simulink library "uavsimBlockset_Cularis_withUAV3D"  (Simulink 8.6)
settings: Solver=ode45  StartTime=0.0  StopTime=10.0  RelTol=1e-3
undefined symbols (not defined in the file): closedloopmask_ID, fflib_degdegm2rrm, flat2lla, uavsim
libraries: uavsimblockset x1, formationFlyingBlockset x1, uavsimBlockset_UAV3DVisualization x1
settings Model: Creator=mstolle  LastModifiedBy=j.bolting

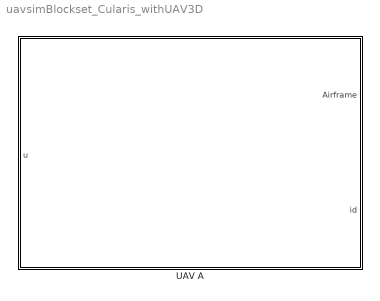
== system uavsimBlockset_Cularis_withUAV3D ==
  UAV A : Subsystem  mask{aircraftmask_phithetapsi0=uavsim.formation(closedloopmask_ID).phithetapsi0, aircraftmask_p0_NED_m=uavsim.formation(closedloopmask_ID).p0_NED', aircraftmask_originNED_ECEF_rrm=uavsim.originNED_ECEF_radradm, aircraftmask_pqr0=uavsim.formation(closedloopmask_ID).omega0, aircraftmask_uvw0=uavsim.formation(closedloopmask_ID).uvw0, aircraftmask_phithetapsi_trim=uavsim.formation(closedloopmask_ID).phithetapsi0, aircraftmask_ID=closedloopmask_ID, aircraftmask_wakevortexenabled=off, aircraftmask_navigationLaw=-1, uavsim=uavsim, leaderID=0, aircraftmask_displayUAV3D=on, aircraftmask_displayVortices=off}
      mask prompts: aircraftmask_phithetapsi0 "Initial Euler angles [rad]"; aircraftmask_p0_NED_m "Initial position, NED frame [m]"; aircraftmask_originNED_ECEF_rrm "Origin NED frame. ECEF, [rad rad m]"; aircraftmask_pqr0 "Initial rotation rates, body frame [rad/s]"; aircraftmask_uvw0 "Initial velocity, body frame [m/s]"; aircraftmask_phithetapsi_trim "Trim Euler angles [rad]"; aircraftmask_ID "Aircraft ID"; aircraftmask_wakevortexenabled "Wake vortex interaction enabled"; aircraftmask_navigationLaw "Active navigation law (-1: automatic selection)"; uavsim "Parameter set"; leaderID "Follows which ID?"; aircraftmask_displayUAV3D "Display in UAV3D"; aircraftmask_displayVortices "Display vortices in UAV3D"
      mask Display:
      | % Set Icon:
      | %image(imread('images/cularis.png'), [.2, .2, .6, .6])

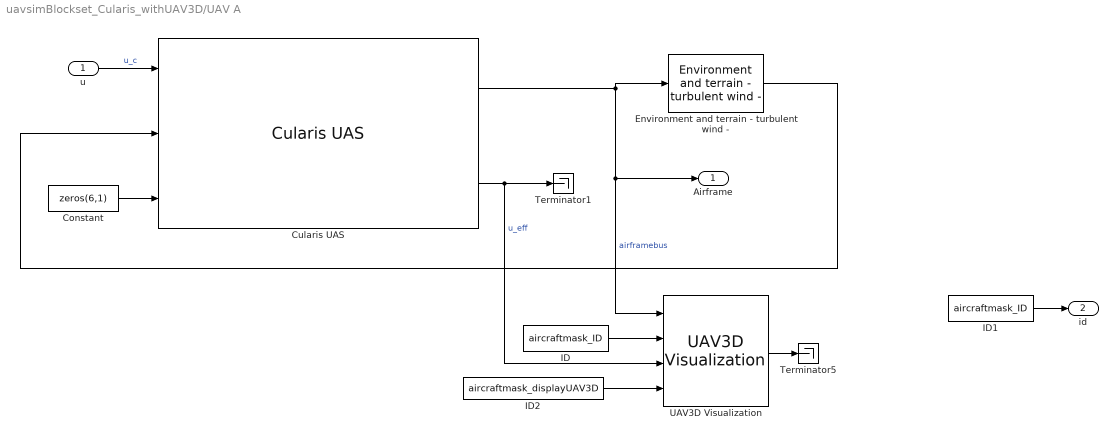
== system uavsimBlockset_Cularis_withUAV3D/UAV A ==
  u : Inport  OutDataTypeStr=Bus: CMD
  Constant : Constant  Value=zeros(6,1)
  Cularis UAS : uavsimblockset/Cularis UAS  mask_cularis_phithetapsi0=aircraftmask_phithetapsi0  mask_cularis_p0_ECEF_lla=fflib_degdegm2rrm(flat2lla(aircraftmask_p0_NED_m, rad2deg(aircraftmask_originNED_ECEF_rrm(1:2)), 0, aircraftmask_originNED_ECEF_rrm(3)))  mask_cularis_originNED_ECEF_rrm=aircraftmask_originNED_ECEF_rrm  mask_cularis_pqr0=aircraftmask_pqr0  mask_cularis_uvw0=aircraftmask_uvw0  uavsim=uavsim
  Environment and terrain - turbulent wind - : formationFlyingBlockset/Environment and terrain - turbulent wind -  mask_ambientWind=uavsim.environment.ambientWind_NED_mps  mask_wingspan=uavsim.cularis.b  mask_turbulenceON=on  mask_windON=on
  ID : Constant  Value=aircraftmask_ID
  ID1 : Constant  Value=aircraftmask_ID
  ID2 : Constant  Value=aircraftmask_displayUAV3D
  Terminator1 : Terminator
  Terminator5 : Terminator
  UAV3D Visualization : uavsimBlockset_UAV3DVisualization/UAV3D Visualization  mask_visual=2
  Airframe : Outport  OutDataTypeStr=Bus: Airframe
  id : Outport  Port=2
  wires:
  Constant/1 -> Cularis UAS/3
  Cularis UAS/1 -> Environment and terrain - turbulent wind -/1, UAV3D Visualization/1, Airframe/1  "airframebus"
  Environment and terrain - turbulent wind -/1 -> Cularis UAS/2
  ID/1 -> UAV3D Visualization/2
  UAV3D Visualization/1 -> Terminator5/1
  u/1 -> Cularis UAS/1  "u_c"
  Cularis UAS/2 -> Terminator1/1, UAV3D Visualization/3  "u_eff"
  ID1/1 -> id/1
  ID2/1 -> UAV3D Visualization/4
